simulink library "pdc_grc"  (R2024a)
settings: Solver=VariableStepAuto  StartTime=0.0  StopTime=10.0  RelTol=1e-3
undefined symbols (not defined in the file or in its folder): ENUM_IVTROPMODE_ASCHI, ENUM_IVTROPMODE_ASCLO, ENUM_IVTROPMODE_DTCYCTRL, ENUM_IVTROPMODE_FW, ENUM_IVTROPMODE_IVTROFF, KASC_DecDuty_value, KASC_OpenTime_s, KCCM_ASCSwitchEna_flg, KDSM_bIvtrTarHiDebug_flg, KDSM_DiagSpdH_rpm, KDSM_DiagSpdL_rpm, KeMCCR_b_UseMeasCrntDTC, KeSVMR_b_UseStrictClamp, KeSVMR_FullDTCCurr_A, KeSVMR_PWMPrd_cnt, KeSVMR_StrClampMaxDuty_pct, KeSVMR_StrClampMinDuty_pct, KeSVMR_t_DeadTime, KeSVMR_t_MinPulseWidth, KOSP_IvtrTarMor_enum_ovrdflg, KOSP_IvtrTarMor_enum_ovrdval, KPDC_facScalePWM_C, KPDC_FWCnt_C, KPDC_nPosnErrMaxSpd_C, StIvtrMod, StMotMod
libraries: simulink x18, GRC_Lib x6
(part 2 of 3)

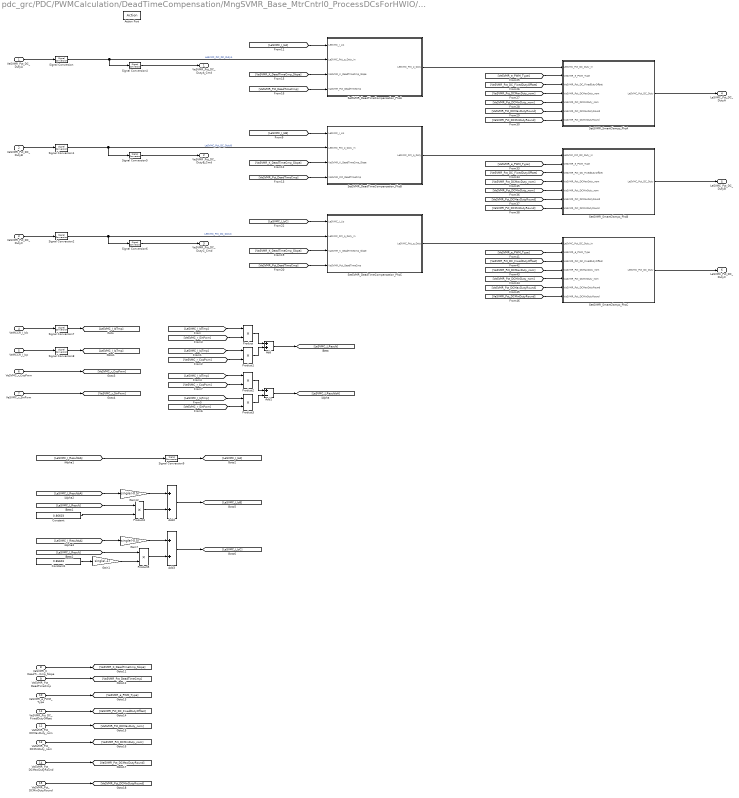
== system pdc_grc/PDC/PWMCalculation/DeadTimeCompensation/MngSVMR_Base_MtrCntrl0_ProcessDCsForHWIO/If Action Subsystem ==
  VeSVMR_Pct_DC_DutyA : Inport
  VeSVMR_Pct_DC_DutyB : Inport  Port=2
  VeSVMR_Pct_DC_DutyC : Inport  Port=3
  VeMCCR_I_Idx : Inport  Port=4
  VeMCCR_I_Iqx : Inport  Port=5
  VeSVMC_r_CosPwm : Inport  Port=6
  VeSVMC_r_SinPwm : Inport  Port=7
  VaSVMR_K_DeadTimeCmp_Slope : Inport  Port=8
  VaSVMR_Pct_DeadTimeCmp : Inport  Port=9
  VeSVMR_e_PWM_Type : Inport  Port=10
  VeSVMR_Pct_DC_FixedDutyOffset : Inport  Port=11
  VaSVMR_Pct_DCMaxDuty_nom : Inport  Port=12
  VaSVMR_Pct_DCMinDuty_nom : Inport  Port=13
  VaSVMR_Pct_DCMaxDutyRound : Inport  Port=14
  VaSVMR_Pct_DCMinDutyRound : Inport  Port=15
  Action Port : ActionPort
  Add : Sum
  Add1 : Sum  Inputs=+-
  Add2 : Sum
  Add3 : Sum
  Constant : Constant  Value=0.86603  OutDataTypeStr=single
      settings: AttributesFormatString=dd_value = 0.86603
  Constant1 : Constant  Value=0.86603  OutDataTypeStr=single
      settings: AttributesFormatString=dd_value = 0.86603
  Gain1 : Gain  Gain=single(-1)
  Gain12 : Gain  Gain=single(-0.5)
  Gain7 : Gain  Gain=single(-0.5)
  Product{,1..5} (6 alike) : Product
  SetSVMR_DeadTimeCompensation_PhsA : Subsystem  TreatAsAtomicUnit=on  RTWFcnName=SetSVMR_DeadTimeCompensation_PhsA  RTWFileName=svmcmbas
      settings: RTWFcnNameOpts=User specified  RTWFileNameOpts=User specified
  SetSVMR_DeadTimeCompensation_PhsB : Subsystem  TreatAsAtomicUnit=on  RTWFcnName=SetSVMR_DeadTimeCompensation_PhsB  RTWFileName=svmcmbas
      settings: RTWFcnNameOpts=User specified  RTWFileNameOpts=User specified
  SetSVMR_DeadTimeCompensation_PhsC : Subsystem  TreatAsAtomicUnit=on  RTWFcnName=SetSVMR_DeadTimeCompensation_PhsC  RTWFileName=svmcmbas
      settings: RTWFcnNameOpts=User specified  RTWFileNameOpts=User specified
  SetSVMR_SmartClamps_PhsA : Subsystem  TreatAsAtomicUnit=on  RTWFcnName=SetSVMR_SmartClamps  RTWFileName=svmcmbas
      settings: RTWFcnNameOpts=User specified  RTWFileNameOpts=User specified
  SetSVMR_SmartClamps_PhsB : Subsystem  TreatAsAtomicUnit=on  RTWFcnName=SetSVMR_SmartClamps  RTWFileName=svmcmbas
      settings: RTWFcnNameOpts=User specified  RTWFileNameOpts=User specified
  SetSVMR_SmartClamps_PhsC : Subsystem  TreatAsAtomicUnit=on  RTWFcnName=SetSVMR_SmartClamps  RTWFileName=svmcmbas
      settings: RTWFcnNameOpts=User specified  RTWFileNameOpts=User specified
  Signal Conversion{,1..2,4..9} (9 alike) : SignalConversion  OverrideOpt=off
  VeSVMR_Pct_DC_DutyA_Cmd : Outport  VectorParamsAs1DForOutWhenUnconnected=off
  VeSVMR_Pct_DC_DutyB_Cmd : Outport  Port=2  VectorParamsAs1DForOutWhenUnconnected=off
  VeSVMR_Pct_DC_DutyC_Cmd : Outport  Port=3  VectorParamsAs1DForOutWhenUnconnected=off
  LeSVMC_Pct_DC_DutyA : Outport  Port=4  VectorParamsAs1DForOutWhenUnconnected=off
  LeSVMC_Pct_DC_DutyB : Outport  Port=5  VectorParamsAs1DForOutWhenUnconnected=off
  LeSVMC_Pct_DC_DutyC : Outport  Port=6  VectorParamsAs1DForOutWhenUnconnected=off
  wires:
  [VeSVMC_r_SinPwm] -> Product/2
  [LeSVMC_I_IsB] -> SetSVMR_DeadTimeCompensation_PhsB/1(LeSVMC_I_Lis)
  SetSVMR_SmartClamps_PhsC/1(LeSVMC_Pct_DC_Duty) -> LeSVMC_Pct_DC_DutyC/1
  SetSVMR_SmartClamps_PhsB/1(LeSVMC_Pct_DC_Duty) -> LeSVMC_Pct_DC_DutyB/1
  SetSVMR_SmartClamps_PhsA/1(LeSVMC_Pct_DC_Duty) -> LeSVMC_Pct_DC_DutyA/1
  [VaSVMR_Pct_DCMinDutyRound] -> SetSVMR_SmartClamps_PhsC/7(VaSVMR_Pct_DCMinDutyRound)
  SetSVMR_DeadTimeCompensation_PhsC/1(LeSVMC_Pct_p_Duty) -> SetSVMR_SmartClamps_PhsC/1(LeSVMC_Pct_DC_Duty_in)
  [VaSVMR_Pct_DCMaxDutyRound] -> SetSVMR_SmartClamps_PhsC/6(VaSVMR_Pct_DCMaxDutyRound)
  [VeSVMR_Pct_DC_FixedDutyOffset] -> SetSVMR_SmartClamps_PhsC/3(VeSVMR_Pct_DC_FixedDutyOffset)
  [VeSVMR_e_PWM_Type] -> SetSVMR_SmartClamps_PhsC/2(VeSVMR_e_PWM_Type)
  [VaSVMR_Pct_DCMaxDuty_nom] -> SetSVMR_SmartClamps_PhsC/4(VaSVMR_Pct_DCMaxDuty_nom)
  [VaSVMR_Pct_DCMinDuty_nom] -> SetSVMR_SmartClamps_PhsC/5(VaSVMR_Pct_DCMinDuty_nom)
  [VaSVMR_Pct_DCMinDutyRound] -> SetSVMR_SmartClamps_PhsB/7(VaSVMR_Pct_DCMinDutyRound)
  SetSVMR_DeadTimeCompensation_PhsB/1(LeSVMC_Pct_p_Duty) -> SetSVMR_SmartClamps_PhsB/1(LeSVMC_Pct_DC_Duty_in)
  [VeSVMR_e_PWM_Type] -> SetSVMR_SmartClamps_PhsB/2(VeSVMR_e_PWM_Type)
  [VaSVMR_Pct_DCMaxDutyRound] -> SetSVMR_SmartClamps_PhsB/6(VaSVMR_Pct_DCMaxDutyRound)
  [VaSVMR_Pct_DCMaxDuty_nom] -> SetSVMR_SmartClamps_PhsB/4(VaSVMR_Pct_DCMaxDuty_nom)
  [VaSVMR_Pct_DCMinDuty_nom] -> SetSVMR_SmartClamps_PhsB/5(VaSVMR_Pct_DCMinDuty_nom)
  [VeSVMR_Pct_DC_FixedDutyOffset] -> SetSVMR_SmartClamps_PhsB/3(VeSVMR_Pct_DC_FixedDutyOffset)
  [VaSVMR_Pct_DCMinDutyRound] -> SetSVMR_SmartClamps_PhsA/7(VaSVMR_Pct_DCMinDutyRound)
  [VaSVMR_Pct_DCMaxDutyRound] -> SetSVMR_SmartClamps_PhsA/6(VaSVMR_Pct_DCMaxDutyRound)
  [VaSVMR_Pct_DCMinDuty_nom] -> SetSVMR_SmartClamps_PhsA/5(VaSVMR_Pct_DCMinDuty_nom)
  [VaSVMR_Pct_DCMaxDuty_nom] -> SetSVMR_SmartClamps_PhsA/4(VaSVMR_Pct_DCMaxDuty_nom)
  [VeSVMR_Pct_DC_FixedDutyOffset] -> SetSVMR_SmartClamps_PhsA/3(VeSVMR_Pct_DC_FixedDutyOffset)
  [VeSVMR_e_PWM_Type] -> SetSVMR_SmartClamps_PhsA/2(VeSVMR_e_PWM_Type)
  VaSVMR_Pct_DCMinDutyRound/1 -> [VaSVMR_Pct_DCMinDutyRound]
  VaSVMR_Pct_DCMaxDutyRound/1 -> [VaSVMR_Pct_DCMaxDutyRound]
  VaSVMR_Pct_DCMinDuty_nom/1 -> [VaSVMR_Pct_DCMinDuty_nom]
  VaSVMR_Pct_DCMaxDuty_nom/1 -> [VaSVMR_Pct_DCMaxDuty_nom]
  VeSVMR_Pct_DC_FixedDutyOffset/1 -> [VeSVMR_Pct_DC_FixedDutyOffset]
  VeSVMR_e_PWM_Type/1 -> [VeSVMR_e_PWM_Type]
  SetSVMR_DeadTimeCompensation_PhsA/1(LeSVMC_Pct_p_Duty) -> SetSVMR_SmartClamps_PhsA/1(LeSVMC_Pct_DC_Duty_in)
  [VaSVMR_Pct_DeadTimeCmp] -> SetSVMR_DeadTimeCompensation_PhsC/4(VaSVMR_Pct_DeadTimeCmp)
  [VaSVMR_K_DeadTimeCmp_Slope] -> SetSVMR_DeadTimeCompensation_PhsC/3(VaSVMR_K_DeadTimeCmp_Slope)
  [LeSVMC_I_IsC] -> SetSVMR_DeadTimeCompensation_PhsC/1(LeSVMC_I_Lis)
  [VaSVMR_Pct_DeadTimeCmp] -> SetSVMR_DeadTimeCompensation_PhsB/4(VaSVMR_Pct_DeadTimeCmp)
  [VaSVMR_K_DeadTimeCmp_Slope] -> SetSVMR_DeadTimeCompensation_PhsB/3(VaSVMR_K_DeadTimeCmp_Slope)
  [VaSVMR_Pct_DeadTimeCmp] -> SetSVMR_DeadTimeCompensation_PhsA/4(VaSVMR_Pct_DeadTimeCmp)
  [VaSVMR_K_DeadTimeCmp_Slope] -> SetSVMR_DeadTimeCompensation_PhsA/3(VaSVMR_K_DeadTimeCmp_Slope)
  VaSVMR_K_DeadTimeCmp_Slope/1 -> [VaSVMR_K_DeadTimeCmp_Slope]
  VaSVMR_Pct_DeadTimeCmp/1 -> [VaSVMR_Pct_DeadTimeCmp]
  [LeSVMC_I_IsA] -> SetSVMR_DeadTimeCompensation_PhsA/1(LeSVMC_I_Lis)
  Gain1/1 -> Product5/2
  Constant1/1 -> Gain1/1
  Constant/1 -> Product4/2
  Add3/1 -> [LeSVMC_I_IsC]
  Signal Conversion9/1 -> [LeSVMC_I_IsA]
  Gain12/1 -> Add2/1
  [LeSVMC_I_ResultIsA] -> Signal Conversion9/1
  Product5/1 -> Add3/2
  Gain7/1 -> Add3/1
  Add2/1 -> [LeSVMC_I_IsB]
  [LeSVMC_I_Result] -> Product5/1
  [LeSVMC_I_ResultIsA] -> Gain7/1
  Product4/1 -> Add2/2
  [LeSVMC_I_ResultIsA] -> Gain12/1
  [LeSVMC_I_Result] -> Product4/1
  Add1/1 -> [LeSVMC_I_ResultIsA]
  Product3/1 -> Add1/2
  Product2/1 -> Add1/1
  [VeSVMC_r_SinPwm] -> Product3/2
  [LeSVMC_I_IqTmp] -> Product3/1
  [VeSVMC_r_CosPwm] -> Product2/2
  [LeSVMC_I_IdTmp] -> Product2/1
  Add/1 -> [LeSVMC_I_Result]
  Product1/1 -> Add/2
  Product/1 -> Add/1
  [VeSVMC_r_CosPwm] -> Product1/2
  [LeSVMC_I_IqTmp] -> Product1/1
  [LeSVMC_I_IdTmp] -> Product/1
  VeSVMC_r_SinPwm/1 -> [VeSVMC_r_SinPwm]
  VeSVMC_r_CosPwm/1 -> [VeSVMC_r_CosPwm]
  Signal Conversion8/1 -> [LeSVMC_I_IqTmp]
  VeMCCR_I_Iqx/1 -> Signal Conversion8/1
  Signal Conversion7/1 -> [LeSVMC_I_IdTmp]
  VeMCCR_I_Idx/1 -> Signal Conversion7/1
  Signal Conversion6/1 -> VeSVMR_Pct_DC_DutyC_Cmd/1
  Signal Conversion5/1 -> VeSVMR_Pct_DC_DutyB_Cmd/1
  Signal Conversion1/1 -> SetSVMR_DeadTimeCompensation_PhsB/2(LeSVMC_Pct_p_Duty_in), Signal Conversion5/1  "LeSVMC_Pct_DC_DutyB"
  Signal Conversion2/1 -> Signal Conversion6/1, SetSVMR_DeadTimeCompensation_PhsC/2(LeSVMC_Pct_p_Duty_in)  "LeSVMC_Pct_DC_DutyC"
  Signal Conversion/1 -> SetSVMR_DeadTimeCompensation_PhsA/2(LeSVMC_Pct_p_Duty_in), Signal Conversion4/1  "LeSVMC_Pct_DC_DutyA"
  Signal Conversion4/1 -> VeSVMR_Pct_DC_DutyA_Cmd/1
  VeSVMR_Pct_DC_DutyC/1 -> Signal Conversion2/1
  VeSVMR_Pct_DC_DutyB/1 -> Signal Conversion1/1
  VeSVMR_Pct_DC_DutyA/1 -> Signal Conversion/1

== system pdc_grc/PDC/PWMCalculation/DeadTimeCompensation/MngSVMR_Base_MtrCntrl0_ProcessDCsForHWIO/If Action Subsystem1 ==
  Action Port : ActionPort
  Constant{4..6,8..10} (6 alike) : Constant  Value=single(0)
      settings: AttributesFormatString=dd_value = 0
  VeSVMR_Pct_DC_DutyA_Cmd : Outport  VectorParamsAs1DForOutWhenUnconnected=off
  VeSVMR_Pct_DC_DutyB_Cmd : Outport  Port=2  VectorParamsAs1DForOutWhenUnconnected=off
  VeSVMR_Pct_DC_DutyC_Cmd : Outport  Port=3  VectorParamsAs1DForOutWhenUnconnected=off
  LeSVMC_Pct_DC_DutyA : Outport  Port=4  VectorParamsAs1DForOutWhenUnconnected=off
  LeSVMC_Pct_DC_DutyB : Outport  Port=5  VectorParamsAs1DForOutWhenUnconnected=off
  LeSVMC_Pct_DC_DutyC : Outport  Port=6  VectorParamsAs1DForOutWhenUnconnected=off
  wires:
  Constant10/1 -> VeSVMR_Pct_DC_DutyC_Cmd/1
  Constant9/1 -> VeSVMR_Pct_DC_DutyB_Cmd/1
  Constant8/1 -> VeSVMR_Pct_DC_DutyA_Cmd/1
  Constant6/1 -> LeSVMC_Pct_DC_DutyC/1
  Constant5/1 -> LeSVMC_Pct_DC_DutyB/1
  Constant4/1 -> LeSVMC_Pct_DC_DutyA/1

== system pdc_grc/PDC/PWMCalculation/DeadTimeCompensation/MngSVMR_Base_MtrCntrl0_ProcessDCsForHWIO/If Action Subsystem5 ==
  LeMCCR_I_TmpIq : Inport
  LeMCCR_I_TmpId : Inport  Port=2
  Action Port : ActionPort
  VeMCCR_I_Iqx : Outport  VectorParamsAs1DForOutWhenUnconnected=off
  VeMCCR_I_Idx : Outport  Port=2  VectorParamsAs1DForOutWhenUnconnected=off
  wires:
  LeMCCR_I_TmpId/1 -> VeMCCR_I_Idx/1
  LeMCCR_I_TmpIq/1 -> VeMCCR_I_Iqx/1

== system pdc_grc/PDC/PWMCalculation/DeadTimeCompensation/MngSVMR_Base_MtrCntrl0_ProcessDCsForHWIO/If Action Subsystem6 ==
  VeMCDR_I_IsqCmd : Inport
  VeMCDR_I_IsdCmd : Inport  Port=2
  Action Port : ActionPort
  VeMCCR_I_Iqx : Outport  VectorParamsAs1DForOutWhenUnconnected=off
  VeMCCR_I_Idx : Outport  Port=2  VectorParamsAs1DForOutWhenUnconnected=off
  wires:
  VeMCDR_I_IsdCmd/1 -> VeMCCR_I_Idx/1
  VeMCDR_I_IsqCmd/1 -> VeMCCR_I_Iqx/1

== system pdc_grc/PDC/PWMCalculation/DeadTimeCompensation/ReInitSVMR_PWM_Modulation/Not_SVPWM_StrictClamp ==
  LeSVMR_f_InvTs : Inport
  Action Port : ActionPort
  Add : Sum
  Add1 : Sum
  Constant : Constant  Value=single(1)
      settings: AttributesFormatString=dd_value = 1
  Constant1 : Constant  Value=KeSVMR_t_MinPulseWidth
      settings: AttributesFormatString=dd_value = 2.2e-06
  Constant2 : Constant  Value=single(1)
      settings: AttributesFormatString=dd_value = 1
  Constant3 : Constant  Value=single(0.5)
      settings: AttributesFormatString=dd_value = 0.5
  Constant4 : Constant  Value=single(0.5)
      settings: AttributesFormatString=dd_value = 0.5
  Constant5 : Constant  Value=KeSVMR_t_DeadTime
      settings: AttributesFormatString=dd_value = 1.8e-06
  Constant6 : Constant  Value=single(0)
      settings: AttributesFormatString=dd_value = 0
  Product : Product
  Product1 : Product
  Product2 : Product
  Signal Conversion : SignalConversion  OverrideOpt=off
  Signal Conversion1 : SignalConversion  OverrideOpt=off
  Subtract : Sum  Inputs=+-
  VeSVMR_Pct_DCMinDuty_nom : Outport  VectorParamsAs1DForOutWhenUnconnected=off
  VeSVMR_Pct_DCMaxDuty_nom : Outport  Port=2  VectorParamsAs1DForOutWhenUnconnected=off
  VeSVMR_Pct_DCMaxDutyRound : Outport  Port=3  VectorParamsAs1DForOutWhenUnconnected=off
  VeSVMR_Pct_DCMinDutyRound : Outport  Port=4  VectorParamsAs1DForOutWhenUnconnected=off
  VeSVMR_Pct_DC_FixedDutyOffset : Outport  Port=5  VectorParamsAs1DForOutWhenUnconnected=off
  wires:
  Product2/1 -> VeSVMR_Pct_DCMinDutyRound/1
  Signal Conversion1/1 -> VeSVMR_Pct_DCMaxDuty_nom/1
  Signal Conversion/1 -> VeSVMR_Pct_DCMinDuty_nom/1
  Constant6/1 -> VeSVMR_Pct_DC_FixedDutyOffset/1
  Product/1 -> Signal Conversion/1, Product2/2, Subtract/2
  Constant4/1 -> Product2/1
  Product1/1 -> VeSVMR_Pct_DCMaxDutyRound/1
  Constant3/1 -> Product1/1
  Add1/1 -> Product1/2
  Subtract/1 -> Signal Conversion1/1, Add1/2
  Constant2/1 -> Add1/1
  Constant/1 -> Subtract/1
  LeSVMR_f_InvTs/1 -> Product/2
  Add/1 -> Product/1
  Constant1/1 -> Add/2
  Constant5/1 -> Add/1

== system pdc_grc/PDC/PWMCalculation/DeadTimeCompensation/ReInitSVMR_PWM_Modulation/SVPWM_StrictClamp ==
  Action Port : ActionPort
  Add : Sum  Inputs=++-
  Constant : Constant  Value=single(1)
      settings: AttributesFormatString=dd_value = 1
  Constant1 : Constant  Value=KeSVMR_StrClampMaxDuty_pct
      settings: AttributesFormatString=dd_value = 1
  Constant2 : Constant  Value=single(0.5)
      settings: AttributesFormatString=dd_value = 0.5
  Constant3 : Constant  Value=KeSVMR_StrClampMinDuty_pct
      settings: AttributesFormatString=dd_value = 0
  Product : Product
  Signal Conversion : SignalConversion  OverrideOpt=off
  Signal Conversion1 : SignalConversion  OverrideOpt=off
  VaSVMR_Pct_DCMinDuty_nom : Outport  VectorParamsAs1DForOutWhenUnconnected=off
  VaSVMR_Pct_DCMaxDuty_nom : Outport  Port=2  VectorParamsAs1DForOutWhenUnconnected=off
  VeSVMR_Pct_DC_FixedDutyOffset : Outport  Port=3  VectorParamsAs1DForOutWhenUnconnected=off
  wires:
  Signal Conversion1/1 -> VaSVMR_Pct_DCMaxDuty_nom/1
  Signal Conversion/1 -> VaSVMR_Pct_DCMinDuty_nom/1
  Product/1 -> VeSVMR_Pct_DC_FixedDutyOffset/1
  Constant2/1 -> Product/2
  Add/1 -> Product/1
  Constant/1 -> Add/3
  Constant1/1 -> Add/2, Signal Conversion1/1
  Constant3/1 -> Add/1, Signal Conversion/1

== system pdc_grc/PDC/PWMCalculation/DeadTimeCompensation/MngSVMR_Base_MtrCntrl0_ProcessDCsForHWIO/If Action Subsystem/SetSVMR_DeadTimeCompensation_PhsA ==
  LeSVMC_I_Lis : Inport
  LeSVMC_Pct_p_Duty_in : Inport  Port=2
  VaSVMR_K_DeadTimeCmp_Slope : Inport  Port=3
  VaSVMR_Pct_DeadTimeCmp : Inport  Port=4
  Constant : Constant  Value=single(0)
      settings: AttributesFormatString=dd_value = 0
  Constant1 : Constant  Value=single(1)
      settings: AttributesFormatString=dd_value = 1
  If : If  IfExpression=u1 ~= 0
  Logical Operator : Logic  AllPortsSameDT=off  OutDataTypeStr=boolean
  Merge : Merge
  Relational Operator : RelationalOperator  Operator=>  OutDataTypeStr=boolean  InputSameDT=off
  Relational Operator1 : RelationalOperator  Operator=<  OutDataTypeStr=boolean  InputSameDT=off
  Signal Conversion1 : SignalConversion  OverrideOpt=off
  Signal Conversion2 : SignalConversion  OverrideOpt=off
  compensate : Subsystem  TreatAsAtomicUnit=on
  no_compensate : Subsystem  TreatAsAtomicUnit=on
  LeSVMC_Pct_p_Duty : Outport  VectorParamsAs1DForOutWhenUnconnected=off
  wires:
  Signal Conversion1/1 -> [LeSVMC_Pct_DC_lduty]
  LeSVMC_Pct_p_Duty_in/1 -> Signal Conversion1/1
  Signal Conversion2/1 -> LeSVMC_Pct_p_Duty/1  "VeSVMR_Pct_DC_DutyA_AfterDTC"
  [LeSVMC_Pct_DC_lduty] -> compensate/1(LeSVMC_Pct_DC_lduty_in)
  [VaSVMR_K_DeadTimeCmp_Slope] -> compensate/2(VaSVMR_K_DeadTimeCmp_Slope)
  LeSVMC_I_Lis/1 -> compensate/3(LeSVMC_I_Lis)
  [VaSVMR_Pct_DeadTimeCmp] -> compensate/4(VaSVMR_Pct_DeadTimeCmp)
  VaSVMR_Pct_DeadTimeCmp/1 -> [VaSVMR_Pct_DeadTimeCmp]
  VaSVMR_K_DeadTimeCmp_Slope/1 -> [VaSVMR_K_DeadTimeCmp_Slope]
  no_compensate/1(LeSVMC_Pct_DC_lduty) -> Merge/2
  compensate/1(LeSVMC_Pct_DC_lduty) -> Merge/1
  [LeSVMC_Pct_DC_lduty] -> no_compensate/1(LeSVMC_Pct_DC_lduty_in)
  [no_compensate] -> no_compensate/Action
  [compensate] -> compensate/Action
  If/2 -> [no_compensate]
  If/1 -> [compensate]
  Logical Operator/1 -> If/1
  Relational Operator1/1 -> Logical Operator/2
  Relational Operator/1 -> Logical Operator/1
  Constant1/1 -> Relational Operator1/2
  Constant/1 -> Relational Operator/2
  [LeSVMC_Pct_DC_lduty] -> Relational Operator/1, Relational Operator1/1
  Merge/1 -> Signal Conversion2/1

== system pdc_grc/PDC/PWMCalculation/DeadTimeCompensation/MngSVMR_Base_MtrCntrl0_ProcessDCsForHWIO/If Action Subsystem/SetSVMR_DeadTimeCompensation_PhsB ==
  LeSVMC_I_Lis : Inport
  LeSVMC_Pct_p_Duty_in : Inport  Port=2
  VaSVMR_K_DeadTimeCmp_Slope : Inport  Port=3
  VaSVMR_Pct_DeadTimeCmp : Inport  Port=4
  Constant : Constant  Value=single(0)
      settings: AttributesFormatString=dd_value = 0
  Constant1 : Constant  Value=single(1)
      settings: AttributesFormatString=dd_value = 1
  If : If  IfExpression=u1 ~= 0
  Logical Operator : Logic  AllPortsSameDT=off  OutDataTypeStr=boolean
  Merge : Merge
  Relational Operator : RelationalOperator  Operator=>  OutDataTypeStr=boolean  InputSameDT=off
  Relational Operator1 : RelationalOperator  Operator=<  OutDataTypeStr=boolean  InputSameDT=off
  Signal Conversion1 : SignalConversion  OverrideOpt=off
  Signal Conversion2 : SignalConversion  OverrideOpt=off
  compensate : Subsystem  TreatAsAtomicUnit=on
  no_compensate : Subsystem  TreatAsAtomicUnit=on
  LeSVMC_Pct_p_Duty : Outport  VectorParamsAs1DForOutWhenUnconnected=off
  wires:
  Merge/1 -> Signal Conversion2/1
  [LeSVMC_Pct_DC_lduty] -> Relational Operator1/1, Relational Operator/1
  Constant/1 -> Relational Operator/2
  Constant1/1 -> Relational Operator1/2
  Relational Operator/1 -> Logical Operator/1
  Relational Operator1/1 -> Logical Operator/2
  Logical Operator/1 -> If/1
  If/1 -> [compensate]
  If/2 -> [no_compensate]
  [compensate] -> compensate/Action
  [no_compensate] -> no_compensate/Action
  [LeSVMC_Pct_DC_lduty] -> no_compensate/1(LeSVMC_Pct_DC_lduty_in)
  compensate/1(LeSVMC_Pct_DC_lduty) -> Merge/1
  no_compensate/1(LeSVMC_Pct_DC_lduty) -> Merge/2
  VaSVMR_K_DeadTimeCmp_Slope/1 -> [VaSVMR_K_DeadTimeCmp_Slope]
  VaSVMR_Pct_DeadTimeCmp/1 -> [VaSVMR_Pct_DeadTimeCmp]
  [VaSVMR_Pct_DeadTimeCmp] -> compensate/4(VaSVMR_Pct_DeadTimeCmp)
  LeSVMC_I_Lis/1 -> compensate/3(LeSVMC_I_Lis)
  [VaSVMR_K_DeadTimeCmp_Slope] -> compensate/2(VaSVMR_K_DeadTimeCmp_Slope)
  [LeSVMC_Pct_DC_lduty] -> compensate/1(LeSVMC_Pct_DC_lduty_in)
  Signal Conversion2/1 -> LeSVMC_Pct_p_Duty/1  "VeSVMR_Pct_DC_DutyB_AfterDTC"
  LeSVMC_Pct_p_Duty_in/1 -> Signal Conversion1/1
  Signal Conversion1/1 -> [LeSVMC_Pct_DC_lduty]

== system pdc_grc/PDC/PWMCalculation/DeadTimeCompensation/MngSVMR_Base_MtrCntrl0_ProcessDCsForHWIO/If Action Subsystem/SetSVMR_DeadTimeCompensation_PhsC ==
  LeSVMC_I_Lis : Inport
  LeSVMC_Pct_p_Duty_in : Inport  Port=2
  VaSVMR_K_DeadTimeCmp_Slope : Inport  Port=3
  VaSVMR_Pct_DeadTimeCmp : Inport  Port=4
  Constant : Constant  Value=single(0)
      settings: AttributesFormatString=dd_value = 0
  Constant1 : Constant  Value=single(1)
      settings: AttributesFormatString=dd_value = 1
  If : If  IfExpression=u1 ~= 0
  Logical Operator : Logic  AllPortsSameDT=off  OutDataTypeStr=boolean
  Merge : Merge
  Relational Operator : RelationalOperator  Operator=>  OutDataTypeStr=boolean  InputSameDT=off
  Relational Operator1 : RelationalOperator  Operator=<  OutDataTypeStr=boolean  InputSameDT=off
  Signal Conversion1 : SignalConversion  OverrideOpt=off
  Signal Conversion2 : SignalConversion  OverrideOpt=off
  compensate : Subsystem  TreatAsAtomicUnit=on
  no_compensate : Subsystem  TreatAsAtomicUnit=on
  LeSVMC_Pct_p_Duty : Outport  VectorParamsAs1DForOutWhenUnconnected=off
  wires:
  Signal Conversion1/1 -> [LeSVMC_Pct_DC_lduty]
  LeSVMC_Pct_p_Duty_in/1 -> Signal Conversion1/1
  Signal Conversion2/1 -> LeSVMC_Pct_p_Duty/1  "VeSVMR_Pct_DC_DutyC_AfterDTC"
  [LeSVMC_Pct_DC_lduty] -> compensate/1(LeSVMC_Pct_DC_lduty_in)
  [VaSVMR_K_DeadTimeCmp_Slope] -> compensate/2(VaSVMR_K_DeadTimeCmp_Slope)
  LeSVMC_I_Lis/1 -> compensate/3(LeSVMC_I_Lis)
  [VaSVMR_Pct_DeadTimeCmp] -> compensate/4(VaSVMR_Pct_DeadTimeCmp)
  VaSVMR_Pct_DeadTimeCmp/1 -> [VaSVMR_Pct_DeadTimeCmp]
  VaSVMR_K_DeadTimeCmp_Slope/1 -> [VaSVMR_K_DeadTimeCmp_Slope]
  no_compensate/1(LeSVMC_Pct_DC_lduty) -> Merge/2
  compensate/1(LeSVMC_Pct_DC_lduty) -> Merge/1
  [LeSVMC_Pct_DC_lduty] -> no_compensate/1(LeSVMC_Pct_DC_lduty_in)
  [no_compensate] -> no_compensate/Action
  [compensate] -> compensate/Action
  If/2 -> [no_compensate]
  If/1 -> [compensate]
  Logical Operator/1 -> If/1
  Relational Operator1/1 -> Logical Operator/2
  Relational Operator/1 -> Logical Operator/1
  Constant1/1 -> Relational Operator1/2
  Constant/1 -> Relational Operator/2
  [LeSVMC_Pct_DC_lduty] -> Relational Operator/1, Relational Operator1/1
  Merge/1 -> Signal Conversion2/1

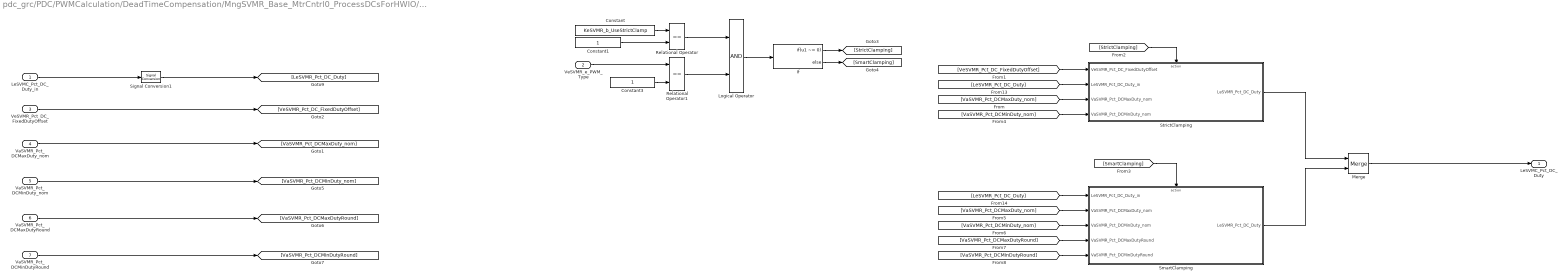
== system pdc_grc/PDC/PWMCalculation/DeadTimeCompensation/MngSVMR_Base_MtrCntrl0_ProcessDCsForHWIO/If Action Subsystem/SetSVMR_SmartClamps_PhsA ==
  LeSVMC_Pct_DC_Duty_in : Inport
  VeSVMR_e_PWM_Type : Inport  Port=2
  VeSVMR_Pct_DC_FixedDutyOffset : Inport  Port=3
  VaSVMR_Pct_DCMaxDuty_nom : Inport  Port=4
  VaSVMR_Pct_DCMinDuty_nom : Inport  Port=5
  VaSVMR_Pct_DCMaxDutyRound : Inport  Port=6
  VaSVMR_Pct_DCMinDutyRound : Inport  Port=7
  Constant : Constant  Value=KeSVMR_b_UseStrictClamp
      settings: AttributesFormatString=dd_value = 0
  Constant1 : Constant
      settings: AttributesFormatString=dd_value = 1
  Constant3 : Constant  OutDataTypeStr=uint8
      settings: AttributesFormatString=dd_value = 1
  If : If  IfExpression=u1 ~= 0
  Logical Operator : Logic  AllPortsSameDT=off  OutDataTypeStr=boolean
  Merge : Merge
  Relational Operator : RelationalOperator  Operator===  OutDataTypeStr=boolean  InputSameDT=off
  Relational Operator1 : RelationalOperator  Operator===  OutDataTypeStr=boolean  InputSameDT=off
  Signal Conversion1 : SignalConversion  OverrideOpt=off
  SmartClamping : Subsystem  TreatAsAtomicUnit=on
  StrictClamping : Subsystem  TreatAsAtomicUnit=on
  LeSVMC_Pct_DC_Duty : Outport  VectorParamsAs1DForOutWhenUnconnected=off
  wires:
  [VaSVMR_Pct_DCMinDutyRound] -> SmartClamping/5(VaSVMR_Pct_DCMinDutyRound)
  [VaSVMR_Pct_DCMaxDutyRound] -> SmartClamping/4(VaSVMR_Pct_DCMaxDutyRound)
  [VaSVMR_Pct_DCMinDuty_nom] -> SmartClamping/3(VaSVMR_Pct_DCMinDuty_nom)
  [VaSVMR_Pct_DCMaxDuty_nom] -> SmartClamping/2(VaSVMR_Pct_DCMaxDuty_nom)
  [VaSVMR_Pct_DCMinDuty_nom] -> StrictClamping/4(VaSVMR_Pct_DCMinDuty_nom)
  [VaSVMR_Pct_DCMaxDuty_nom] -> StrictClamping/3(VaSVMR_Pct_DCMaxDuty_nom)
  Signal Conversion1/1 -> [LeSVMR_Pct_DC_Duty]
  LeSVMC_Pct_DC_Duty_in/1 -> Signal Conversion1/1
  Merge/1 -> LeSVMC_Pct_DC_Duty/1
  SmartClamping/1(LeSVMR_Pct_DC_Duty) -> Merge/2
  StrictClamping/1(LeSVMR_Pct_DC_Duty) -> Merge/1
  [LeSVMR_Pct_DC_Duty] -> SmartClamping/1(LeSVMR_Pct_DC_Duty_in)
  [LeSVMR_Pct_DC_Duty] -> StrictClamping/2(LeSVMR_Pct_DC_Duty_in)
  VaSVMR_Pct_DCMinDutyRound/1 -> [VaSVMR_Pct_DCMinDutyRound]
  VaSVMR_Pct_DCMaxDutyRound/1 -> [VaSVMR_Pct_DCMaxDutyRound]
  VaSVMR_Pct_DCMinDuty_nom/1 -> [VaSVMR_Pct_DCMinDuty_nom]
  [VeSVMR_Pct_DC_FixedDutyOffset] -> StrictClamping/1(VeSVMR_Pct_DC_FixedDutyOffset)
  [SmartClamping] -> SmartClamping/Action
  [StrictClamping] -> StrictClamping/Action
  If/2 -> [SmartClamping]
  If/1 -> [StrictClamping]
  VeSVMR_Pct_DC_FixedDutyOffset/1 -> [VeSVMR_Pct_DC_FixedDutyOffset]
  VaSVMR_Pct_DCMaxDuty_nom/1 -> [VaSVMR_Pct_DCMaxDuty_nom]
  Logical Operator/1 -> If/1
  Relational Operator1/1 -> Logical Operator/2
  Relational Operator/1 -> Logical Operator/1
  Constant3/1 -> Relational Operator1/2
  VeSVMR_e_PWM_Type/1 -> Relational Operator1/1
  Constant1/1 -> Relational Operator/2
  Constant/1 -> Relational Operator/1

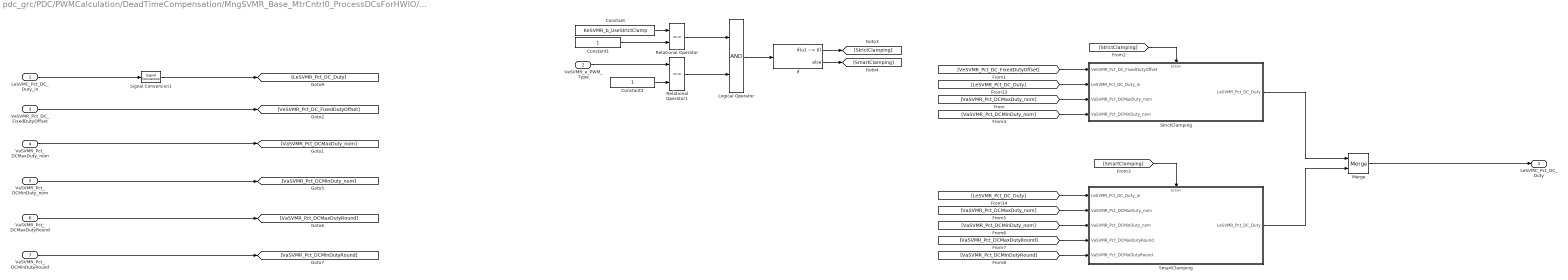
== system pdc_grc/PDC/PWMCalculation/DeadTimeCompensation/MngSVMR_Base_MtrCntrl0_ProcessDCsForHWIO/If Action Subsystem/SetSVMR_SmartClamps_PhsB ==
  LeSVMC_Pct_DC_Duty_in : Inport
  VeSVMR_e_PWM_Type : Inport  Port=2
  VeSVMR_Pct_DC_FixedDutyOffset : Inport  Port=3
  VaSVMR_Pct_DCMaxDuty_nom : Inport  Port=4
  VaSVMR_Pct_DCMinDuty_nom : Inport  Port=5
  VaSVMR_Pct_DCMaxDutyRound : Inport  Port=6
  VaSVMR_Pct_DCMinDutyRound : Inport  Port=7
  Constant : Constant  Value=KeSVMR_b_UseStrictClamp
      settings: AttributesFormatString=dd_value = 0
  Constant1 : Constant
      settings: AttributesFormatString=dd_value = 1
  Constant3 : Constant  OutDataTypeStr=uint8
      settings: AttributesFormatString=dd_value = 1
  If : If  IfExpression=u1 ~= 0
  Logical Operator : Logic  AllPortsSameDT=off  OutDataTypeStr=boolean
  Merge : Merge
  Relational Operator : RelationalOperator  Operator===  OutDataTypeStr=boolean  InputSameDT=off
  Relational Operator1 : RelationalOperator  Operator===  OutDataTypeStr=boolean  InputSameDT=off
  Signal Conversion1 : SignalConversion  OverrideOpt=off
  SmartClamping : Subsystem  TreatAsAtomicUnit=on
  StrictClamping : Subsystem  TreatAsAtomicUnit=on
  LeSVMC_Pct_DC_Duty : Outport  VectorParamsAs1DForOutWhenUnconnected=off
  wires:
  Constant/1 -> Relational Operator/1
  Constant1/1 -> Relational Operator/2
  VeSVMR_e_PWM_Type/1 -> Relational Operator1/1
  Constant3/1 -> Relational Operator1/2
  Relational Operator/1 -> Logical Operator/1
  Relational Operator1/1 -> Logical Operator/2
  Logical Operator/1 -> If/1
  VaSVMR_Pct_DCMaxDuty_nom/1 -> [VaSVMR_Pct_DCMaxDuty_nom]
  VeSVMR_Pct_DC_FixedDutyOffset/1 -> [VeSVMR_Pct_DC_FixedDutyOffset]
  If/1 -> [StrictClamping]
  If/2 -> [SmartClamping]
  [StrictClamping] -> StrictClamping/Action
  [SmartClamping] -> SmartClamping/Action
  [VeSVMR_Pct_DC_FixedDutyOffset] -> StrictClamping/1(VeSVMR_Pct_DC_FixedDutyOffset)
  VaSVMR_Pct_DCMinDuty_nom/1 -> [VaSVMR_Pct_DCMinDuty_nom]
  VaSVMR_Pct_DCMaxDutyRound/1 -> [VaSVMR_Pct_DCMaxDutyRound]
  VaSVMR_Pct_DCMinDutyRound/1 -> [VaSVMR_Pct_DCMinDutyRound]
  [LeSVMR_Pct_DC_Duty] -> StrictClamping/2(LeSVMR_Pct_DC_Duty_in)
  [LeSVMR_Pct_DC_Duty] -> SmartClamping/1(LeSVMR_Pct_DC_Duty_in)
  StrictClamping/1(LeSVMR_Pct_DC_Duty) -> Merge/1
  SmartClamping/1(LeSVMR_Pct_DC_Duty) -> Merge/2
  Merge/1 -> LeSVMC_Pct_DC_Duty/1
  LeSVMC_Pct_DC_Duty_in/1 -> Signal Conversion1/1
  Signal Conversion1/1 -> [LeSVMR_Pct_DC_Duty]
  [VaSVMR_Pct_DCMaxDuty_nom] -> StrictClamping/3(VaSVMR_Pct_DCMaxDuty_nom)
  [VaSVMR_Pct_DCMinDuty_nom] -> StrictClamping/4(VaSVMR_Pct_DCMinDuty_nom)
  [VaSVMR_Pct_DCMaxDuty_nom] -> SmartClamping/2(VaSVMR_Pct_DCMaxDuty_nom)
  [VaSVMR_Pct_DCMinDuty_nom] -> SmartClamping/3(VaSVMR_Pct_DCMinDuty_nom)
  [VaSVMR_Pct_DCMaxDutyRound] -> SmartClamping/4(VaSVMR_Pct_DCMaxDutyRound)
  [VaSVMR_Pct_DCMinDutyRound] -> SmartClamping/5(VaSVMR_Pct_DCMinDutyRound)

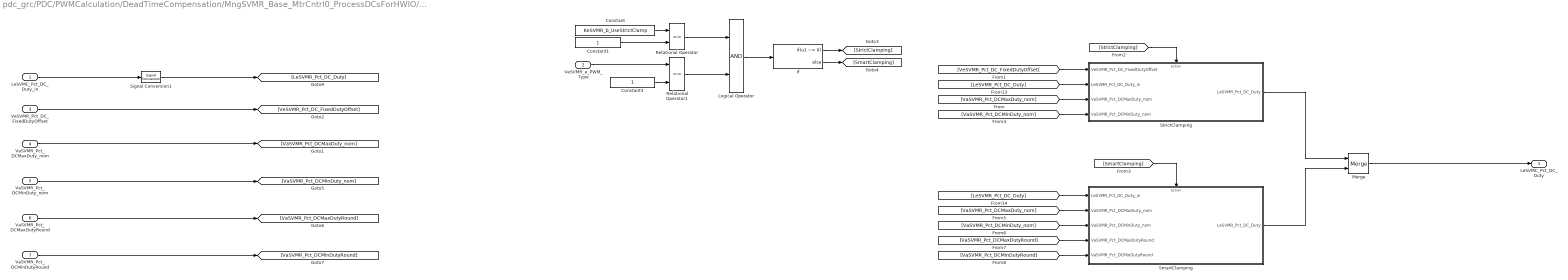
== system pdc_grc/PDC/PWMCalculation/DeadTimeCompensation/MngSVMR_Base_MtrCntrl0_ProcessDCsForHWIO/If Action Subsystem/SetSVMR_SmartClamps_PhsC ==
  LeSVMC_Pct_DC_Duty_in : Inport
  VeSVMR_e_PWM_Type : Inport  Port=2
  VeSVMR_Pct_DC_FixedDutyOffset : Inport  Port=3
  VaSVMR_Pct_DCMaxDuty_nom : Inport  Port=4
  VaSVMR_Pct_DCMinDuty_nom : Inport  Port=5
  VaSVMR_Pct_DCMaxDutyRound : Inport  Port=6
  VaSVMR_Pct_DCMinDutyRound : Inport  Port=7
  Constant : Constant  Value=KeSVMR_b_UseStrictClamp
      settings: AttributesFormatString=dd_value = 0
  Constant1 : Constant
      settings: AttributesFormatString=dd_value = 1
  Constant3 : Constant  OutDataTypeStr=uint8
      settings: AttributesFormatString=dd_value = 1
  If : If  IfExpression=u1 ~= 0
  Logical Operator : Logic  AllPortsSameDT=off  OutDataTypeStr=boolean
  Merge : Merge
  Relational Operator : RelationalOperator  Operator===  OutDataTypeStr=boolean  InputSameDT=off
  Relational Operator1 : RelationalOperator  Operator===  OutDataTypeStr=boolean  InputSameDT=off
  Signal Conversion1 : SignalConversion  OverrideOpt=off
  SmartClamping : Subsystem  TreatAsAtomicUnit=on
  StrictClamping : Subsystem  TreatAsAtomicUnit=on
  LeSVMC_Pct_DC_Duty : Outport  VectorParamsAs1DForOutWhenUnconnected=off
  wires:
  [VaSVMR_Pct_DCMinDutyRound] -> SmartClamping/5(VaSVMR_Pct_DCMinDutyRound)
  [VaSVMR_Pct_DCMaxDutyRound] -> SmartClamping/4(VaSVMR_Pct_DCMaxDutyRound)
  [VaSVMR_Pct_DCMinDuty_nom] -> SmartClamping/3(VaSVMR_Pct_DCMinDuty_nom)
  [VaSVMR_Pct_DCMaxDuty_nom] -> SmartClamping/2(VaSVMR_Pct_DCMaxDuty_nom)
  [VaSVMR_Pct_DCMinDuty_nom] -> StrictClamping/4(VaSVMR_Pct_DCMinDuty_nom)
  [VaSVMR_Pct_DCMaxDuty_nom] -> StrictClamping/3(VaSVMR_Pct_DCMaxDuty_nom)
  Signal Conversion1/1 -> [LeSVMR_Pct_DC_Duty]
  LeSVMC_Pct_DC_Duty_in/1 -> Signal Conversion1/1
  Merge/1 -> LeSVMC_Pct_DC_Duty/1
  SmartClamping/1(LeSVMR_Pct_DC_Duty) -> Merge/2
  StrictClamping/1(LeSVMR_Pct_DC_Duty) -> Merge/1
  [LeSVMR_Pct_DC_Duty] -> SmartClamping/1(LeSVMR_Pct_DC_Duty_in)
  [LeSVMR_Pct_DC_Duty] -> StrictClamping/2(LeSVMR_Pct_DC_Duty_in)
  VaSVMR_Pct_DCMinDutyRound/1 -> [VaSVMR_Pct_DCMinDutyRound]
  VaSVMR_Pct_DCMaxDutyRound/1 -> [VaSVMR_Pct_DCMaxDutyRound]
  VaSVMR_Pct_DCMinDuty_nom/1 -> [VaSVMR_Pct_DCMinDuty_nom]
  [VeSVMR_Pct_DC_FixedDutyOffset] -> StrictClamping/1(VeSVMR_Pct_DC_FixedDutyOffset)
  [SmartClamping] -> SmartClamping/Action
  [StrictClamping] -> StrictClamping/Action
  If/2 -> [SmartClamping]
  If/1 -> [StrictClamping]
  VeSVMR_Pct_DC_FixedDutyOffset/1 -> [VeSVMR_Pct_DC_FixedDutyOffset]
  VaSVMR_Pct_DCMaxDuty_nom/1 -> [VaSVMR_Pct_DCMaxDuty_nom]
  Logical Operator/1 -> If/1
  Relational Operator1/1 -> Logical Operator/2
  Relational Operator/1 -> Logical Operator/1
  Constant3/1 -> Relational Operator1/2
  VeSVMR_e_PWM_Type/1 -> Relational Operator1/1
  Constant1/1 -> Relational Operator/2
  Constant/1 -> Relational Operator/1

== system pdc_grc/PDC/PWMCalculation/DeadTimeCompensation/MngSVMR_Base_MtrCntrl0_ProcessDCsForHWIO/If Action Subsystem/SetSVMR_DeadTimeCompensation_PhsA/compensate ==
  LeSVMC_Pct_DC_lduty_in : Inport
  VaSVMR_K_DeadTimeCmp_Slope : Inport  Port=2
  LeSVMC_I_Lis : Inport  Port=3
  VaSVMR_Pct_DeadTimeCmp : Inport  Port=4
  Action Port : ActionPort
  Add : Sum
  Gain : Gain  Gain=single(-1)
  Product : Product
  Relational Operator : RelationalOperator  Operator=>  OutDataTypeStr=boolean  InputSameDT=off
  Relational Operator1 : RelationalOperator  Operator=<  OutDataTypeStr=boolean  InputSameDT=off
  Switch : Switch  Criteria=u2 ~= 0  SaturateOnIntegerOverflow=off  InputSameDT=off
  Switch1 : Switch  Criteria=u2 ~= 0  SaturateOnIntegerOverflow=off  InputSameDT=off
  LeSVMC_Pct_DC_lduty : Outport  VectorParamsAs1DForOutWhenUnconnected=off
  wires:
  VaSVMR_Pct_DeadTimeCmp/1 -> [LaSVMR_Pct_DeadTimeCmp_PeriodIndex]
  VaSVMR_K_DeadTimeCmp_Slope/1 -> Product/1
  Add/1 -> LeSVMC_Pct_DC_lduty/1
  LeSVMC_Pct_DC_lduty_in/1 -> Add/1
  Switch/1 -> Add/2
  [LeSVMC_Pct_DeadTimeCmp] -> Switch1/3
  Relational Operator1/1 -> Switch1/2
  [LaSVMR_Pct_DeadTimeCmp_PeriodIndex] -> Gain/1
  Gain/1 -> Relational Operator1/2, Switch1/1
  [LeSVMC_Pct_DeadTimeCmp] -> Relational Operator1/1
  Switch1/1 -> Switch/3
  [LaSVMR_Pct_DeadTimeCmp_PeriodIndex] -> Switch/1
  Relational Operator/1 -> Switch/2
  [LaSVMR_Pct_DeadTimeCmp_PeriodIndex] -> Relational Operator/2
  [LeSVMC_Pct_DeadTimeCmp] -> Relational Operator/1
  Product/1 -> [LeSVMC_Pct_DeadTimeCmp]
  LeSVMC_I_Lis/1 -> Product/2

== system pdc_grc/PDC/PWMCalculation/DeadTimeCompensation/MngSVMR_Base_MtrCntrl0_ProcessDCsForHWIO/If Action Subsystem/SetSVMR_DeadTimeCompensation_PhsA/no_compensate ==
  LeSVMC_Pct_DC_lduty_in : Inport
  Action Port : ActionPort
  Signal Conversion : SignalConversion  OverrideOpt=off
  LeSVMC_Pct_DC_lduty : Outport  VectorParamsAs1DForOutWhenUnconnected=off
  wires:
  Signal Conversion/1 -> LeSVMC_Pct_DC_lduty/1
  LeSVMC_Pct_DC_lduty_in/1 -> Signal Conversion/1

== system pdc_grc/PDC/PWMCalculation/DeadTimeCompensation/MngSVMR_Base_MtrCntrl0_ProcessDCsForHWIO/If Action Subsystem/SetSVMR_DeadTimeCompensation_PhsB/compensate ==
  LeSVMC_Pct_DC_lduty_in : Inport
  VaSVMR_K_DeadTimeCmp_Slope : Inport  Port=2
  LeSVMC_I_Lis : Inport  Port=3
  VaSVMR_Pct_DeadTimeCmp : Inport  Port=4
  Action Port : ActionPort
  Add : Sum
  Gain : Gain  Gain=single(-1)
  Product : Product
  Relational Operator : RelationalOperator  Operator=>  OutDataTypeStr=boolean  InputSameDT=off
  Relational Operator1 : RelationalOperator  Operator=<  OutDataTypeStr=boolean  InputSameDT=off
  Switch : Switch  Criteria=u2 ~= 0  SaturateOnIntegerOverflow=off  InputSameDT=off
  Switch1 : Switch  Criteria=u2 ~= 0  SaturateOnIntegerOverflow=off  InputSameDT=off
  LeSVMC_Pct_DC_lduty : Outport  VectorParamsAs1DForOutWhenUnconnected=off
  wires:
  LeSVMC_I_Lis/1 -> Product/2
  Product/1 -> [LeSVMC_Pct_DeadTimeCmp]
  [LeSVMC_Pct_DeadTimeCmp] -> Relational Operator/1
  [LaSVMR_Pct_DeadTimeCmp_PeriodIndex] -> Relational Operator/2
  Relational Operator/1 -> Switch/2
  [LaSVMR_Pct_DeadTimeCmp_PeriodIndex] -> Switch/1
  Switch1/1 -> Switch/3
  [LeSVMC_Pct_DeadTimeCmp] -> Relational Operator1/1
  Gain/1 -> Switch1/1, Relational Operator1/2
  [LaSVMR_Pct_DeadTimeCmp_PeriodIndex] -> Gain/1
  Relational Operator1/1 -> Switch1/2
  [LeSVMC_Pct_DeadTimeCmp] -> Switch1/3
  Switch/1 -> Add/2
  LeSVMC_Pct_DC_lduty_in/1 -> Add/1
  Add/1 -> LeSVMC_Pct_DC_lduty/1
  VaSVMR_K_DeadTimeCmp_Slope/1 -> Product/1
  VaSVMR_Pct_DeadTimeCmp/1 -> [LaSVMR_Pct_DeadTimeCmp_PeriodIndex]

== system pdc_grc/PDC/PWMCalculation/DeadTimeCompensation/MngSVMR_Base_MtrCntrl0_ProcessDCsForHWIO/If Action Subsystem/SetSVMR_DeadTimeCompensation_PhsB/no_compensate ==
  LeSVMC_Pct_DC_lduty_in : Inport
  Action Port : ActionPort
  Signal Conversion : SignalConversion  OverrideOpt=off
  LeSVMC_Pct_DC_lduty : Outport  VectorParamsAs1DForOutWhenUnconnected=off
  wires:
  LeSVMC_Pct_DC_lduty_in/1 -> Signal Conversion/1
  Signal Conversion/1 -> LeSVMC_Pct_DC_lduty/1

== system pdc_grc/PDC/PWMCalculation/DeadTimeCompensation/MngSVMR_Base_MtrCntrl0_ProcessDCsForHWIO/If Action Subsystem/SetSVMR_DeadTimeCompensation_PhsC/compensate ==
  LeSVMC_Pct_DC_lduty_in : Inport
  VaSVMR_K_DeadTimeCmp_Slope : Inport  Port=2
  LeSVMC_I_Lis : Inport  Port=3
  VaSVMR_Pct_DeadTimeCmp : Inport  Port=4
  Action Port : ActionPort
  Add : Sum
  Gain : Gain  Gain=single(-1)
  Product : Product
  Relational Operator : RelationalOperator  Operator=>  OutDataTypeStr=boolean  InputSameDT=off
  Relational Operator1 : RelationalOperator  Operator=<  OutDataTypeStr=boolean  InputSameDT=off
  Switch : Switch  Criteria=u2 ~= 0  SaturateOnIntegerOverflow=off  InputSameDT=off
  Switch1 : Switch  Criteria=u2 ~= 0  SaturateOnIntegerOverflow=off  InputSameDT=off
  LeSVMC_Pct_DC_lduty : Outport  VectorParamsAs1DForOutWhenUnconnected=off
  wires:
  VaSVMR_Pct_DeadTimeCmp/1 -> [LaSVMR_Pct_DeadTimeCmp_PeriodIndex]
  VaSVMR_K_DeadTimeCmp_Slope/1 -> Product/1
  Add/1 -> LeSVMC_Pct_DC_lduty/1
  LeSVMC_Pct_DC_lduty_in/1 -> Add/1
  Switch/1 -> Add/2
  [LeSVMC_Pct_DeadTimeCmp] -> Switch1/3
  Relational Operator1/1 -> Switch1/2
  [LaSVMR_Pct_DeadTimeCmp_PeriodIndex] -> Gain/1
  Gain/1 -> Relational Operator1/2, Switch1/1
  [LeSVMC_Pct_DeadTimeCmp] -> Relational Operator1/1
  Switch1/1 -> Switch/3
  [LaSVMR_Pct_DeadTimeCmp_PeriodIndex] -> Switch/1
  Relational Operator/1 -> Switch/2
  [LaSVMR_Pct_DeadTimeCmp_PeriodIndex] -> Relational Operator/2
  [LeSVMC_Pct_DeadTimeCmp] -> Relational Operator/1
  Product/1 -> [LeSVMC_Pct_DeadTimeCmp]
  LeSVMC_I_Lis/1 -> Product/2

== system pdc_grc/PDC/PWMCalculation/DeadTimeCompensation/MngSVMR_Base_MtrCntrl0_ProcessDCsForHWIO/If Action Subsystem/SetSVMR_DeadTimeCompensation_PhsC/no_compensate ==
  LeSVMC_Pct_DC_lduty_in : Inport
  Action Port : ActionPort
  Signal Conversion : SignalConversion  OverrideOpt=off
  LeSVMC_Pct_DC_lduty : Outport  VectorParamsAs1DForOutWhenUnconnected=off
  wires:
  Signal Conversion/1 -> LeSVMC_Pct_DC_lduty/1
  LeSVMC_Pct_DC_lduty_in/1 -> Signal Conversion/1

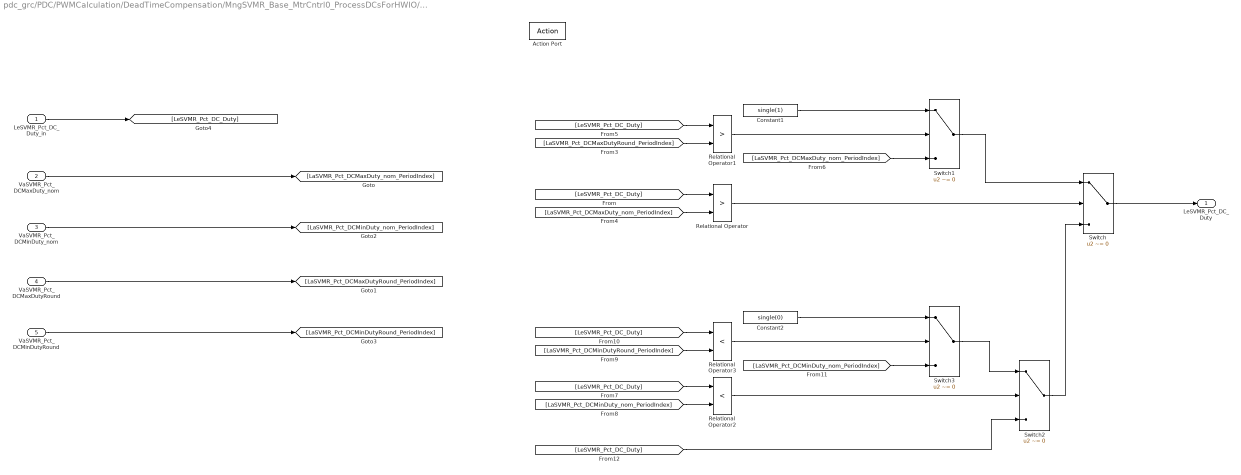
== system pdc_grc/PDC/PWMCalculation/DeadTimeCompensation/MngSVMR_Base_MtrCntrl0_ProcessDCsForHWIO/If Action Subsystem/SetSVMR_SmartClamps_PhsA/SmartClamping ==
  LeSVMR_Pct_DC_Duty_in : Inport
  VaSVMR_Pct_DCMaxDuty_nom : Inport  Port=2
  VaSVMR_Pct_DCMinDuty_nom : Inport  Port=3
  VaSVMR_Pct_DCMaxDutyRound : Inport  Port=4
  VaSVMR_Pct_DCMinDutyRound : Inport  Port=5
  Action Port : ActionPort
  Constant1 : Constant  Value=single(1)
      settings: AttributesFormatString=dd_value = 1
  Constant2 : Constant  Value=single(0)
      settings: AttributesFormatString=dd_value = 0
  Relational Operator : RelationalOperator  Operator=>  OutDataTypeStr=boolean  InputSameDT=off
  Relational Operator1 : RelationalOperator  Operator=>  OutDataTypeStr=boolean  InputSameDT=off
  Relational Operator2 : RelationalOperator  Operator=<  OutDataTypeStr=boolean  InputSameDT=off
  Relational Operator3 : RelationalOperator  Operator=<  OutDataTypeStr=boolean  InputSameDT=off
  Switch{,1..3} (4 alike) : Switch  Criteria=u2 ~= 0  SaturateOnIntegerOverflow=off  InputSameDT=off
  LeSVMR_Pct_DC_Duty : Outport  VectorParamsAs1DForOutWhenUnconnected=off
  wires:
  VaSVMR_Pct_DCMaxDutyRound/1 -> [LaSVMR_Pct_DCMaxDutyRound_PeriodIndex]
  VaSVMR_Pct_DCMinDuty_nom/1 -> [LaSVMR_Pct_DCMinDuty_nom_PeriodIndex]
  Switch/1 -> LeSVMR_Pct_DC_Duty/1
  [LeSVMR_Pct_DC_Duty] -> Switch2/3
  [LaSVMR_Pct_DCMinDuty_nom_PeriodIndex] -> Switch3/3
  Constant2/1 -> Switch3/1
  Switch3/1 -> Switch2/1
  Switch2/1 -> Switch/3
  Relational Operator3/1 -> Switch3/2
  [LaSVMR_Pct_DCMinDutyRound_PeriodIndex] -> Relational Operator3/2
  [LeSVMR_Pct_DC_Duty] -> Relational Operator3/1
  Relational Operator2/1 -> Switch2/2
  [LaSVMR_Pct_DCMinDuty_nom_PeriodIndex] -> Relational Operator2/2
  [LeSVMR_Pct_DC_Duty] -> Relational Operator2/1
  Switch1/1 -> Switch/1
  [LaSVMR_Pct_DCMaxDuty_nom_PeriodIndex] -> Switch1/3
  Constant1/1 -> Switch1/1
  Relational Operator1/1 -> Switch1/2
  [LaSVMR_Pct_DCMaxDutyRound_PeriodIndex] -> Relational Operator1/2
  [LeSVMR_Pct_DC_Duty] -> Relational Operator1/1
  Relational Operator/1 -> Switch/2
  [LaSVMR_Pct_DCMaxDuty_nom_PeriodIndex] -> Relational Operator/2
  [LeSVMR_Pct_DC_Duty] -> Relational Operator/1
  LeSVMR_Pct_DC_Duty_in/1 -> [LeSVMR_Pct_DC_Duty]
  VaSVMR_Pct_DCMinDutyRound/1 -> [LaSVMR_Pct_DCMinDutyRound_PeriodIndex]
  VaSVMR_Pct_DCMaxDuty_nom/1 -> [LaSVMR_Pct_DCMaxDuty_nom_PeriodIndex]

== system pdc_grc/PDC/PWMCalculation/DeadTimeCompensation/MngSVMR_Base_MtrCntrl0_ProcessDCsForHWIO/If Action Subsystem/SetSVMR_SmartClamps_PhsA/StrictClamping ==
  VeSVMR_Pct_DC_FixedDutyOffset : Inport
  LeSVMR_Pct_DC_Duty_in : Inport  Port=2
  VaSVMR_Pct_DCMaxDuty_nom : Inport  Port=3
  VaSVMR_Pct_DCMinDuty_nom : Inport  Port=4
  Action Port : ActionPort
  Add : Sum
  Relational Operator : RelationalOperator  Operator=>  OutDataTypeStr=boolean  InputSameDT=off
  Relational Operator1 : RelationalOperator  Operator=<  OutDataTypeStr=boolean  InputSameDT=off
  Switch : Switch  Criteria=u2 ~= 0  SaturateOnIntegerOverflow=off  InputSameDT=off
  Switch2 : Switch  Criteria=u2 ~= 0  SaturateOnIntegerOverflow=off  InputSameDT=off
  LeSVMR_Pct_DC_Duty : Outport  VectorParamsAs1DForOutWhenUnconnected=off
  wires:
  VaSVMR_Pct_DCMinDuty_nom/1 -> [LaSVMR_Pct_DCMinDuty_nom_PeriodIndex]
  [LaSVMR_Pct_DCMaxDuty_nom_PeriodIndex] -> Relational Operator/2
  VaSVMR_Pct_DCMaxDuty_nom/1 -> [LaSVMR_Pct_DCMaxDuty_nom_PeriodIndex]
  Switch/1 -> LeSVMR_Pct_DC_Duty/1
  [LeSVMR_Pct_DC_Duty] -> Switch2/3
  [LaSVMR_Pct_DCMinDuty_nom_PeriodIndex] -> Switch2/1
  Relational Operator1/1 -> Switch2/2
  [LaSVMR_Pct_DCMinDuty_nom_PeriodIndex] -> Relational Operator1/2
  [LeSVMR_Pct_DC_Duty] -> Relational Operator1/1
  Switch2/1 -> Switch/3
  [LaSVMR_Pct_DCMaxDuty_nom_PeriodIndex] -> Switch/1
  Relational Operator/1 -> Switch/2
  [LeSVMR_Pct_DC_Duty] -> Relational Operator/1
  Add/1 -> [LeSVMR_Pct_DC_Duty]
  LeSVMR_Pct_DC_Duty_in/1 -> Add/2
  VeSVMR_Pct_DC_FixedDutyOffset/1 -> Add/1

== system pdc_grc/PDC/PWMCalculation/DeadTimeCompensation/MngSVMR_Base_MtrCntrl0_ProcessDCsForHWIO/If Action Subsystem/SetSVMR_SmartClamps_PhsB/SmartClamping ==
  LeSVMR_Pct_DC_Duty_in : Inport
  VaSVMR_Pct_DCMaxDuty_nom : Inport  Port=2
  VaSVMR_Pct_DCMinDuty_nom : Inport  Port=3
  VaSVMR_Pct_DCMaxDutyRound : Inport  Port=4
  VaSVMR_Pct_DCMinDutyRound : Inport  Port=5
  Action Port : ActionPort
  Constant1 : Constant  Value=single(1)
      settings: AttributesFormatString=dd_value = 1
  Constant2 : Constant  Value=single(0)
      settings: AttributesFormatString=dd_value = 0
  Relational Operator : RelationalOperator  Operator=>  OutDataTypeStr=boolean  InputSameDT=off
  Relational Operator1 : RelationalOperator  Operator=>  OutDataTypeStr=boolean  InputSameDT=off
  Relational Operator2 : RelationalOperator  Operator=<  OutDataTypeStr=boolean  InputSameDT=off
  Relational Operator3 : RelationalOperator  Operator=<  OutDataTypeStr=boolean  InputSameDT=off
  Switch{,1..3} (4 alike) : Switch  Criteria=u2 ~= 0  SaturateOnIntegerOverflow=off  InputSameDT=off
  LeSVMR_Pct_DC_Duty : Outport  VectorParamsAs1DForOutWhenUnconnected=off
  wires:
  VaSVMR_Pct_DCMaxDuty_nom/1 -> [LaSVMR_Pct_DCMaxDuty_nom_PeriodIndex]
  VaSVMR_Pct_DCMinDutyRound/1 -> [LaSVMR_Pct_DCMinDutyRound_PeriodIndex]
  LeSVMR_Pct_DC_Duty_in/1 -> [LeSVMR_Pct_DC_Duty]
  [LeSVMR_Pct_DC_Duty] -> Relational Operator/1
  [LaSVMR_Pct_DCMaxDuty_nom_PeriodIndex] -> Relational Operator/2
  Relational Operator/1 -> Switch/2
  [LeSVMR_Pct_DC_Duty] -> Relational Operator1/1
  [LaSVMR_Pct_DCMaxDutyRound_PeriodIndex] -> Relational Operator1/2
  Relational Operator1/1 -> Switch1/2
  Constant1/1 -> Switch1/1
  [LaSVMR_Pct_DCMaxDuty_nom_PeriodIndex] -> Switch1/3
  Switch1/1 -> Switch/1
  [LeSVMR_Pct_DC_Duty] -> Relational Operator2/1
  [LaSVMR_Pct_DCMinDuty_nom_PeriodIndex] -> Relational Operator2/2
  Relational Operator2/1 -> Switch2/2
  [LeSVMR_Pct_DC_Duty] -> Relational Operator3/1
  [LaSVMR_Pct_DCMinDutyRound_PeriodIndex] -> Relational Operator3/2
  Relational Operator3/1 -> Switch3/2
  Switch2/1 -> Switch/3
  Switch3/1 -> Switch2/1
  Constant2/1 -> Switch3/1
  [LaSVMR_Pct_DCMinDuty_nom_PeriodIndex] -> Switch3/3
  [LeSVMR_Pct_DC_Duty] -> Switch2/3
  Switch/1 -> LeSVMR_Pct_DC_Duty/1
  VaSVMR_Pct_DCMinDuty_nom/1 -> [LaSVMR_Pct_DCMinDuty_nom_PeriodIndex]
  VaSVMR_Pct_DCMaxDutyRound/1 -> [LaSVMR_Pct_DCMaxDutyRound_PeriodIndex]

== system pdc_grc/PDC/PWMCalculation/DeadTimeCompensation/MngSVMR_Base_MtrCntrl0_ProcessDCsForHWIO/If Action Subsystem/SetSVMR_SmartClamps_PhsB/StrictClamping ==
  VeSVMR_Pct_DC_FixedDutyOffset : Inport
  LeSVMR_Pct_DC_Duty_in : Inport  Port=2
  VaSVMR_Pct_DCMaxDuty_nom : Inport  Port=3
  VaSVMR_Pct_DCMinDuty_nom : Inport  Port=4
  Action Port : ActionPort
  Add : Sum
  Relational Operator : RelationalOperator  Operator=>  OutDataTypeStr=boolean  InputSameDT=off
  Relational Operator1 : RelationalOperator  Operator=<  OutDataTypeStr=boolean  InputSameDT=off
  Switch : Switch  Criteria=u2 ~= 0  SaturateOnIntegerOverflow=off  InputSameDT=off
  Switch2 : Switch  Criteria=u2 ~= 0  SaturateOnIntegerOverflow=off  InputSameDT=off
  LeSVMR_Pct_DC_Duty : Outport  VectorParamsAs1DForOutWhenUnconnected=off
  wires:
  VeSVMR_Pct_DC_FixedDutyOffset/1 -> Add/1
  LeSVMR_Pct_DC_Duty_in/1 -> Add/2
  Add/1 -> [LeSVMR_Pct_DC_Duty]
  [LeSVMR_Pct_DC_Duty] -> Relational Operator/1
  Relational Operator/1 -> Switch/2
  [LaSVMR_Pct_DCMaxDuty_nom_PeriodIndex] -> Switch/1
  Switch2/1 -> Switch/3
  [LeSVMR_Pct_DC_Duty] -> Relational Operator1/1
  [LaSVMR_Pct_DCMinDuty_nom_PeriodIndex] -> Relational Operator1/2
  Relational Operator1/1 -> Switch2/2
  [LaSVMR_Pct_DCMinDuty_nom_PeriodIndex] -> Switch2/1
  [LeSVMR_Pct_DC_Duty] -> Switch2/3
  Switch/1 -> LeSVMR_Pct_DC_Duty/1
  VaSVMR_Pct_DCMaxDuty_nom/1 -> [LaSVMR_Pct_DCMaxDuty_nom_PeriodIndex]
  [LaSVMR_Pct_DCMaxDuty_nom_PeriodIndex] -> Relational Operator/2
  VaSVMR_Pct_DCMinDuty_nom/1 -> [LaSVMR_Pct_DCMinDuty_nom_PeriodIndex]

== system pdc_grc/PDC/PWMCalculation/DeadTimeCompensation/MngSVMR_Base_MtrCntrl0_ProcessDCsForHWIO/If Action Subsystem/SetSVMR_SmartClamps_PhsC/SmartClamping ==
  LeSVMR_Pct_DC_Duty_in : Inport
  VaSVMR_Pct_DCMaxDuty_nom : Inport  Port=2
  VaSVMR_Pct_DCMinDuty_nom : Inport  Port=3
  VaSVMR_Pct_DCMaxDutyRound : Inport  Port=4
  VaSVMR_Pct_DCMinDutyRound : Inport  Port=5
  Action Port : ActionPort
  Constant1 : Constant  Value=single(1)
      settings: AttributesFormatString=dd_value = 1
  Constant2 : Constant  Value=single(0)
      settings: AttributesFormatString=dd_value = 0
  Relational Operator : RelationalOperator  Operator=>  OutDataTypeStr=boolean  InputSameDT=off
  Relational Operator1 : RelationalOperator  Operator=>  OutDataTypeStr=boolean  InputSameDT=off
  Relational Operator2 : RelationalOperator  Operator=<  OutDataTypeStr=boolean  InputSameDT=off
  Relational Operator3 : RelationalOperator  Operator=<  OutDataTypeStr=boolean  InputSameDT=off
  Switch{,1..3} (4 alike) : Switch  Criteria=u2 ~= 0  SaturateOnIntegerOverflow=off  InputSameDT=off
  LeSVMR_Pct_DC_Duty : Outport  VectorParamsAs1DForOutWhenUnconnected=off
  wires:
  VaSVMR_Pct_DCMaxDutyRound/1 -> [LaSVMR_Pct_DCMaxDutyRound_PeriodIndex]
  VaSVMR_Pct_DCMinDuty_nom/1 -> [LaSVMR_Pct_DCMinDuty_nom_PeriodIndex]
  Switch/1 -> LeSVMR_Pct_DC_Duty/1
  [LeSVMR_Pct_DC_Duty] -> Switch2/3
  [LaSVMR_Pct_DCMinDuty_nom_PeriodIndex] -> Switch3/3
  Constant2/1 -> Switch3/1
  Switch3/1 -> Switch2/1
  Switch2/1 -> Switch/3
  Relational Operator3/1 -> Switch3/2
  [LaSVMR_Pct_DCMinDutyRound_PeriodIndex] -> Relational Operator3/2
  [LeSVMR_Pct_DC_Duty] -> Relational Operator3/1
  Relational Operator2/1 -> Switch2/2
  [LaSVMR_Pct_DCMinDuty_nom_PeriodIndex] -> Relational Operator2/2
  [LeSVMR_Pct_DC_Duty] -> Relational Operator2/1
  Switch1/1 -> Switch/1
  [LaSVMR_Pct_DCMaxDuty_nom_PeriodIndex] -> Switch1/3
  Constant1/1 -> Switch1/1
  Relational Operator1/1 -> Switch1/2
  [LaSVMR_Pct_DCMaxDutyRound_PeriodIndex] -> Relational Operator1/2
  [LeSVMR_Pct_DC_Duty] -> Relational Operator1/1
  Relational Operator/1 -> Switch/2
  [LaSVMR_Pct_DCMaxDuty_nom_PeriodIndex] -> Relational Operator/2
  [LeSVMR_Pct_DC_Duty] -> Relational Operator/1
  LeSVMR_Pct_DC_Duty_in/1 -> [LeSVMR_Pct_DC_Duty]
  VaSVMR_Pct_DCMinDutyRound/1 -> [LaSVMR_Pct_DCMinDutyRound_PeriodIndex]
  VaSVMR_Pct_DCMaxDuty_nom/1 -> [LaSVMR_Pct_DCMaxDuty_nom_PeriodIndex]

== system pdc_grc/PDC/PWMCalculation/DeadTimeCompensation/MngSVMR_Base_MtrCntrl0_ProcessDCsForHWIO/If Action Subsystem/SetSVMR_SmartClamps_PhsC/StrictClamping ==
  VeSVMR_Pct_DC_FixedDutyOffset : Inport
  LeSVMR_Pct_DC_Duty_in : Inport  Port=2
  VaSVMR_Pct_DCMaxDuty_nom : Inport  Port=3
  VaSVMR_Pct_DCMinDuty_nom : Inport  Port=4
  Action Port : ActionPort
  Add : Sum
  Relational Operator : RelationalOperator  Operator=>  OutDataTypeStr=boolean  InputSameDT=off
  Relational Operator1 : RelationalOperator  Operator=<  OutDataTypeStr=boolean  InputSameDT=off
  Switch : Switch  Criteria=u2 ~= 0  SaturateOnIntegerOverflow=off  InputSameDT=off
  Switch2 : Switch  Criteria=u2 ~= 0  SaturateOnIntegerOverflow=off  InputSameDT=off
  LeSVMR_Pct_DC_Duty : Outport  VectorParamsAs1DForOutWhenUnconnected=off
  wires:
  VaSVMR_Pct_DCMinDuty_nom/1 -> [LaSVMR_Pct_DCMinDuty_nom_PeriodIndex]
  [LaSVMR_Pct_DCMaxDuty_nom_PeriodIndex] -> Relational Operator/2
  VaSVMR_Pct_DCMaxDuty_nom/1 -> [LaSVMR_Pct_DCMaxDuty_nom_PeriodIndex]
  Switch/1 -> LeSVMR_Pct_DC_Duty/1
  [LeSVMR_Pct_DC_Duty] -> Switch2/3
  [LaSVMR_Pct_DCMinDuty_nom_PeriodIndex] -> Switch2/1
  Relational Operator1/1 -> Switch2/2
  [LaSVMR_Pct_DCMinDuty_nom_PeriodIndex] -> Relational Operator1/2
  [LeSVMR_Pct_DC_Duty] -> Relational Operator1/1
  Switch2/1 -> Switch/3
  [LaSVMR_Pct_DCMaxDuty_nom_PeriodIndex] -> Switch/1
  Relational Operator/1 -> Switch/2
  [LeSVMR_Pct_DC_Duty] -> Relational Operator/1
  Add/1 -> [LeSVMR_Pct_DC_Duty]
  LeSVMR_Pct_DC_Duty_in/1 -> Add/2
  VeSVMR_Pct_DC_FixedDutyOffset/1 -> Add/1
